simulink model "testIMU"  (R2021a)
settings: Solver=VariableStepAuto  StartTime=0.0  StopTime=10  RelTol=1e-3
libraries: simulink x6
settings Model: Creator=jmher  LastModifiedBy=jmher

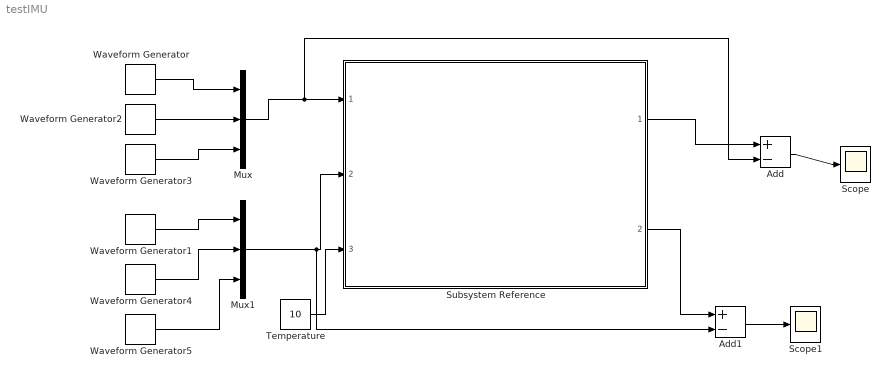
== system testIMU ==
  Add : Sum  Inputs=+-
  Add1 : Sum  Inputs=+-
  Mux : Mux  Inputs=3
  Mux1 : Mux  Inputs=3
  Scope : Scope
  Scope1 : Scope
  Subsystem Reference : Subsystem  ReferencedSubsystem=IMU
  Temperature : Constant  Value=10
  Waveform Generator : simulink/Sources/Waveform Generator  OutMin=[]  OutMax=[]  OutDataTypeStr=double  SelectedSignal=1  Signals=sin(1,0.5,0)  BlockNames=MultiportSwitch_3e06f62d4adc469  SampleTime=0.001
  Waveform Generator1 : simulink/Sources/Waveform Generator  OutMin=[]  OutMax=[]  OutDataTypeStr=double  SelectedSignal=1  Signals=sin(0.1,0.5,0)  BlockNames=MultiportSwitch_16dbc7e0913e4d9  SampleTime=0.001
  Waveform Generator2 : simulink/Sources/Waveform Generator  OutMin=[]  OutMax=[]  OutDataTypeStr=double  SelectedSignal=1  Signals=sin(1,0.5,0)  BlockNames=MultiportSwitch_41985427b8c94e8  SampleTime=0.001
  Waveform Generator3 : simulink/Sources/Waveform Generator  OutMin=[]  OutMax=[]  OutDataTypeStr=double  SelectedSignal=1  Signals=sin(1,0.5,0)  BlockNames=MultiportSwitch_96e4d37e10e2487  SampleTime=0.001
  Waveform Generator4 : simulink/Sources/Waveform Generator  OutMin=[]  OutMax=[]  OutDataTypeStr=double  SelectedSignal=1  Signals=sin(0.1,0.5,0)  BlockNames=MultiportSwitch_b591075ed67e4dd  SampleTime=0.001
  Waveform Generator5 : simulink/Sources/Waveform Generator  OutMin=[]  OutMax=[]  OutDataTypeStr=double  SelectedSignal=1  Signals=sin(0.1,0.5,0)  BlockNames=MultiportSwitch_88b78efc1abf426  SampleTime=0.001
  wires:
  Subsystem Reference/1 -> Add/1
  Mux/1 -> Add/2, Subsystem Reference/1
  Waveform Generator3/1 -> Mux/3
  Waveform Generator2/1 -> Mux/2
  Waveform Generator/1 -> Mux/1
  Mux1/1 -> Add1/2, Subsystem Reference/2
  Waveform Generator1/1 -> Mux1/1
  Waveform Generator4/1 -> Mux1/2
  Waveform Generator5/1 -> Mux1/3
  Temperature/1 -> Subsystem Reference/3
  Add/1 -> Scope/1
  Subsystem Reference/2 -> Add1/1
  Add1/1 -> Scope1/1
